simulink model "VCU_CS75_12_30_test"  (R2014a)
settings: Solver=FixedStepDiscrete  StartTime=0.0  StopTime=25  FixedStep=0.0005  RelTol=1e-3
InitFcn:
  | PID_canshu
values from neighbouring files (symbols this model uses):
  D1 = ecucoder_cal(D1)    [PID_canshu.m]
  D2 = ecucoder_cal(D2)    [PID_canshu.m]
  D3 = ecucoder_cal(D3)    [PID_canshu.m]
  ErrorLimit = ecucoder_cal(ErrorLimit)    [PID_canshu.m]
  ErrorSumMax1 = ecucoder_cal(ErrorSumMax1)    [PID_canshu.m]
  ErrorSumMax2 = ecucoder_cal(ErrorSumMax2)    [PID_canshu.m]
  ErrorSumMax3 = ecucoder_cal(ErrorSumMax3)    [PID_canshu.m]
  I1 = ecucoder_cal(I1)    [PID_canshu.m]
  I2 = ecucoder_cal(I2)    [PID_canshu.m]
  I3 = ecucoder_cal(I3)    [PID_canshu.m]
  Limit1 = ecucoder_cal(Limit1)    [PID_canshu.m]
  Limit2 = ecucoder_cal(Limit2)    [PID_canshu.m]
  P1 = ecucoder_cal(P1)    [PID_canshu.m]
  P2 = ecucoder_cal(P2)    [PID_canshu.m]
  P3 = ecucoder_cal(P3)    [PID_canshu.m]
  T_buchang = ecucoder_cal(T_buchang)    [PID_canshu.m]
undefined symbols (not defined in the file or in its folder): ecucoder_acal, I_SW01_L, LaterlAngleCommand, LDW, RemoteAcclPosition
libraries: simulink x940, ec5744lib x41
(part 13 of 31)

== system VCU_CS75_12_30_test/长安CS75底盘程序，20ms一次/Input/CAN1_Rx/GW_3A2/ReceiveMessages/Subsystem ==
  input : Inport
  Enable : EnablePort
  Bus Creator : BusCreator  Inputs=27
  GW_3A1 : Subsystem
  Signal Conversion : SignalConversion
  GW_3A2 : Outport
  wires:
  input/1 -> GW_3A1/1(input)
  Bus Creator/1 -> Signal Conversion/1
  GW_3A1/1(EPS_TorqueAssistMode_Out) -> Bus Creator/1  "EPS_TorqueAssistMode"
  GW_3A1/2(EMS_RemindGear_Out) -> Bus Creator/2  "EMS_RemindGear"
  GW_3A1/3(TCU_FailureLamp_Out) -> Bus Creator/3  "TCU_FailureLamp"
  GW_3A1/4(ACC_ACCMode_Out) -> Bus Creator/4  "ACC_ACCMode"
  GW_3A1/5(TCU_WNTLamp_Out) -> Bus Creator/5  "TCU_WNTLamp"
  GW_3A1/6(TCU_PWRLamp_Out) -> Bus Creator/6  "TCU_PWRLamp"
  GW_3A1/7(SRS_LeftRearBuckleSwitchSts_Out) -> Bus Creator/7  "SRS_LeftRearBuckleSwitchSts"
  GW_3A1/8(SRS_MiddleRearBuckleSwitchSts_Out) -> Bus Creator/8  "SRS_MiddleRearBuckleSwitchSts"
  GW_3A1/9(SRS_RightRearBuckleSwitchSts_Out) -> Bus Creator/9  "SRS_RightRearBuckleSwitchSts"
  GW_3A1/10(EPB_TextDisplay_Out) -> Bus Creator/10  "EPB_TextDisplay"
  GW_3A1/11(ESP_ESPActiveStatus_Out) -> Bus Creator/11  "ESP_ESPActiveStatus"
  GW_3A1/12(ESP_ESPFunctionStatus_Out) -> Bus Creator/12  "ESP_ESPFunctionStatus"
  GW_3A1/13(ESP_EBDFailStatus_Out) -> Bus Creator/13  "ESP_EBDFailStatus"
  GW_3A1/14(EPS_EPSFailed_Out) -> Bus Creator/14  "EPS_EPSFailed"
  GW_3A1/15(EPB_FunctionLamp_Out) -> Bus Creator/15  "EPB_FunctionLamp"
  GW_3A1/16(EPB_SwitchPosition_Out) -> Bus Creator/16  "EPB_SwitchPosition"
  GW_3A1/17(EPB_SwitchPositionValid_Out) -> Bus Creator/17  "EPB_SwitchPositionValid"
  GW_3A1/18(ESP_HDC_STATUS_Out) -> Bus Creator/18  "ESP_HDC_STATUS"
  GW_3A1/19(ESP_AutoHoldAvailable_Out) -> Bus Creator/19  "ESP_AutoHoldAvailable"
  GW_3A1/20(ESP_HHC_Active_Out) -> Bus Creator/20  "ESP_HHC_Active"
  GW_3A1/21(ESP_AutoHoldActive_Out) -> Bus Creator/21  "ESP_AutoHoldActive"
  GW_3A1/22(ESP_HHC_Available_Out) -> Bus Creator/22  "ESP_HHC_Available"
  GW_3A1/23(TCU_GearForDisplay_Out) -> Bus Creator/23  "TCU_GearForDisplay"
  GW_3A1/24(ESP_HBBFunctionStatus_Out) -> Bus Creator/24  "ESP_HBBFunctionStatus"
  GW_3A1/25(TCU_GearIndication_Out) -> Bus Creator/25  "TCU_GearIndication"
  GW_3A1/26(TCU_ReqTranTempWarning_Out) -> Bus Creator/26  "TCU_ReqTranTempWarning"
  GW_3A1/27(EMS_RemindShiftGear_Out) -> Bus Creator/27  "EMS_RemindShiftGear"
  Signal Conversion/1 -> GW_3A2/1

== system VCU_CS75_12_30_test/长安CS75底盘程序，20ms一次/Input/CAN1_Rx/GW_567/ReceiveMessages/Subsystem ==
  input : Inport
  Enable : EnablePort
  Bus Creator : BusCreator  Inputs=5
  GW_2 : Subsystem
  Signal Conversion : SignalConversion
  GW_567 : Outport
  wires:
  Bus Creator/1 -> Signal Conversion/1
  input/1 -> GW_2/1(input)
  GW_2/1(HU_EnterTunnelInfo_Out) -> Bus Creator/1  "HU_EnterTunnelInfo"
  GW_2/2(HU_TunnelDistance_Out) -> Bus Creator/2  "HU_TunnelDistance"
  GW_2/3(HU_TunnelLength_Out) -> Bus Creator/3  "HU_TunnelLength"
  GW_2/4(HU_Byroad_Out) -> Bus Creator/4  "HU_Byroad"
  GW_2/5(HU_NavGuiganceStatus_Out) -> Bus Creator/5  "HU_NavGuiganceStatus"
  Signal Conversion/1 -> GW_567/1

== system VCU_CS75_12_30_test/长安CS75底盘程序，20ms一次/Input/CAN1_Rx/HU_GPS_500/ReceiveMessages/Subsystem ==
  input : Inport
  Enable : EnablePort
  Bus Creator : BusCreator  Inputs=1
  HU_GPS_1 : Subsystem
  Signal Conversion : SignalConversion
  HU_GPS_500 : Outport
  wires:
  input/1 -> HU_GPS_1/1(input)
  Bus Creator/1 -> Signal Conversion/1
  HU_GPS_1/1(GPSCurrentLocationValid_Out) -> Bus Creator/1  "GPSCurrentLocationValid"
  Signal Conversion/1 -> HU_GPS_500/1

== system VCU_CS75_12_30_test/长安CS75底盘程序，20ms一次/Input/CAN1_Rx/LAS_36E/ReceiveMessages/Subsystem ==
  input : Inport
  Enable : EnablePort
  Bus Creator : BusCreator  Inputs=7
  LAS_36E2 : Subsystem
  Signal Conversion : SignalConversion
  LAS_36E : Outport
  wires:
  Bus Creator/1 -> Signal Conversion/1
  input/1 -> LAS_36E2/1(input)
  LAS_36E2/1(LAS_RoadCurvatureFar_Out) -> Bus Creator/1  "LAS_RoadCurvatureFar"
  LAS_36E2/2(LAS_RoadCurvatureNear_Out) -> Bus Creator/2  "LAS_RoadCurvatureNear"
  LAS_36E2/3(LAS_LaneEquationC1_Out) -> Bus Creator/3  "LAS_LaneEquationC1"
  LAS_36E2/4(LAS_LaneEquationC3_Out) -> Bus Creator/4  "LAS_LaneEquationC3"
  LAS_36E2/5(LAS_RollingCounter_id36E_Out) -> Bus Creator/5  "LAS_RollingCounter_id36E"
  LAS_36E2/6(LAS_LaneEquationStatus_Out) -> Bus Creator/6  "LAS_LaneEquationStatus"
  LAS_36E2/7(LAS_CheckSum_id36E_Out) -> Bus Creator/7  "LAS_CheckSum_id36E"
  Signal Conversion/1 -> LAS_36E/1

== system VCU_CS75_12_30_test/长安CS75底盘程序，20ms一次/Input/CAN1_Rx/SAS_108/ReceiveMessages/Subsystem ==
  input : Inport
  Enable : EnablePort
  Bus Creator : BusCreator  Inputs=7
  SAS_2 : Subsystem
  Signal Conversion : SignalConversion
  SAS_108 : Outport
  wires:
  Bus Creator/1 -> Signal Conversion/1
  input/1 -> SAS_2/1(input)
  SAS_2/1(SAS_SteeringAngle_Out) -> Bus Creator/1  "SAS_SteeringAngle"
  SAS_2/2(SAS_SteeringAngleSpeed_Out) -> Bus Creator/2  "SAS_SteeringAngleSpeed"
  SAS_2/3(SAS_Calibrated_Out) -> Bus Creator/3  "SAS_Calibrated"
  SAS_2/4(SAS_SASFailure_Out) -> Bus Creator/4  "SAS_SASFailure"
  SAS_2/5(SAS_SteeringAngleValid_Out) -> Bus Creator/5  "SAS_SteeringAngleValid"
  SAS_2/6(SAS_RollingCounter_Out) -> Bus Creator/6  "SAS_RollingCounter"
  SAS_2/7(SAS_CRCCheck_Out) -> Bus Creator/7  "SAS_CRCCheck"
  Signal Conversion/1 -> SAS_108/1

== system VCU_CS75_12_30_test/长安CS75底盘程序，20ms一次/Input/CAN1_Rx/SCM_3B8/ReceiveMessages/Subsystem ==
  input : Inport
  Enable : EnablePort
  Bus Creator : BusCreator  Inputs=6
  SCM_3B2 : Subsystem
  Signal Conversion : SignalConversion
  SCM_3B8 : Outport
  wires:
  input/1 -> SCM_3B2/1(input)
  Bus Creator/1 -> Signal Conversion/1
  SCM_3B2/6(SCM_IACCOn_Out) -> Bus Creator/6  "SCM_IACCOn"
  SCM_3B2/5(SCM_TimeGap_Out) -> Bus Creator/5  "SCM_TimeGap"
  SCM_3B2/4(SCM_Speeddecrease_Out) -> Bus Creator/4  "SCM_Speeddecrease"
  SCM_3B2/3(SCM_Resume_Out) -> Bus Creator/3  "SCM_Resume"
  SCM_3B2/2(SCM_ACCCancel_Out) -> Bus Creator/2  "SCM_ACCCancel"
  SCM_3B2/1(SCM_ACCOn_Out) -> Bus Creator/1  "SCM_ACCOn"
  Signal Conversion/1 -> SCM_3B8/1

== system VCU_CS75_12_30_test/长安CS75底盘程序，20ms一次/Input/CAN1_Rx/SRS_005/ReceiveMessages/Subsystem ==
  input : Inport
  Enable : EnablePort
  Bus Creator : BusCreator  Inputs=2
  SRS_1 : Subsystem
  Signal Conversion : SignalConversion
  SRS_005 : Outport
  wires:
  Bus Creator/1 -> Signal Conversion/1
  input/1 -> SRS_1/1(input)
  SRS_1/1(SRS_DriverBuckleSwitchStatus_Out) -> Bus Creator/1  "SRS_DriverBuckleSwitchStatus"
  SRS_1/2(SRS_RollingCounter_Out) -> Bus Creator/2  "SRS_RollingCounter"
  Signal Conversion/1 -> SRS_005/1

== system VCU_CS75_12_30_test/长安CS75底盘程序，20ms一次/Input/CAN1_Rx/TCU_286/ReceiveMessages/Subsystem ==
  input : Inport
  Enable : EnablePort
  Bus Creator : BusCreator
  Signal Conversion : SignalConversion
  TCU_1 : Subsystem
  TCU_286 : Outport
  wires:
  input/1 -> TCU_1/1(input)
  Bus Creator/1 -> Signal Conversion/1
  TCU_1/1(TCU_ActualGear_Out) -> Bus Creator/1  "TCU_ActualGear"
  TCU_1/2(TCU_ShiftPositionValid_Out) -> Bus Creator/2  "TCU_ShiftPositionValid"
  TCU_1/3(TCU_ActualGearValid_Out) -> Bus Creator/3  "TCU_ActualGearValid"
  TCU_1/4(TCU_GearShiftPosition_Out) -> Bus Creator/4  "TCU_GearShiftPosition"
  Signal Conversion/1 -> TCU_286/1

== system VCU_CS75_12_30_test/长安CS75底盘程序，20ms一次/Input/DBC转化的messages（存底）/ReceiveMessages/EMS_205/EMS_CheckSum_205_Sub ==
  In1 : Inport
  Out1 : Outport
  wires:
  In1/1 -> Out1/1

== system VCU_CS75_12_30_test/长安CS75底盘程序，20ms一次/Input/DBC转化的messages（存底）/ReceiveMessages/EMS_205/EMS_ESPTorqReuestAvailability_Sub ==
  In1 : Inport
  Out1 : Outport
  wires:
  In1/1 -> Out1/1

== system VCU_CS75_12_30_test/长安CS75底盘程序，20ms一次/Input/DBC转化的messages（存底）/ReceiveMessages/EMS_205/EMS_FrictionalTorq_Sub ==
  In1 : Inport
  Out1 : Outport
  wires:
  In1/1 -> Out1/1

== system VCU_CS75_12_30_test/长安CS75底盘程序，20ms一次/Input/DBC转化的messages（存底）/ReceiveMessages/EMS_205/EMS_IndicatedDriverReqTorq_Sub ==
  In1 : Inport
  Out1 : Outport
  wires:
  In1/1 -> Out1/1

== system VCU_CS75_12_30_test/长安CS75底盘程序，20ms一次/Input/DBC转化的messages（存底）/ReceiveMessages/EMS_205/EMS_IndicatedRealEngTorq_Sub ==
  In1 : Inport
  Out1 : Outport
  wires:
  In1/1 -> Out1/1

== system VCU_CS75_12_30_test/长安CS75底盘程序，20ms一次/Input/DBC转化的messages（存底）/ReceiveMessages/EMS_205/EMS_RollingCounter_id205_Sub ==
  In1 : Inport
  Out1 : Outport
  wires:
  In1/1 -> Out1/1

== system VCU_CS75_12_30_test/长安CS75底盘程序，20ms一次/Input/DBC转化的messages（存底）/ReceiveMessages/EMS_205/EMS_TorqFailure_Sub ==
  In1 : Inport
  Out1 : Outport
  wires:
  In1/1 -> Out1/1

== system VCU_CS75_12_30_test/长安CS75底盘程序，20ms一次/Input/DBC转化的messages（存底）/ReceiveMessages1/EMS_255/EMS_AccPedal_Sub ==
  In1 : Inport
  Out1 : Outport
  wires:
  In1/1 -> Out1/1

== system VCU_CS75_12_30_test/长安CS75底盘程序，20ms一次/Input/DBC转化的messages（存底）/ReceiveMessages1/EMS_255/EMS_AccpedelError_Sub ==
  In1 : Inport
  Out1 : Outport
  wires:
  In1/1 -> Out1/1

== system VCU_CS75_12_30_test/长安CS75底盘程序，20ms一次/Input/DBC转化的messages（存底）/ReceiveMessages1/EMS_255/EMS_BrakePedalStatus_Sub ==
  In1 : Inport
  Out1 : Outport
  wires:
  In1/1 -> Out1/1

== system VCU_CS75_12_30_test/长安CS75底盘程序，20ms一次/Input/DBC转化的messages（存底）/ReceiveMessages1/EMS_255/EMS_CheckSum_255_Sub ==
  In1 : Inport
  Out1 : Outport
  wires:
  In1/1 -> Out1/1

== system VCU_CS75_12_30_test/长安CS75底盘程序，20ms一次/Input/DBC转化的messages（存底）/ReceiveMessages1/EMS_255/EMS_EngineSpeedError_Sub ==
  In1 : Inport
  Out1 : Outport
  wires:
  In1/1 -> Out1/1

== system VCU_CS75_12_30_test/长安CS75底盘程序，20ms一次/Input/DBC转化的messages（存底）/ReceiveMessages1/EMS_255/EMS_EngineSpeed_Sub ==
  In1 : Inport
  Out1 : Outport
  wires:
  In1/1 -> Out1/1

== system VCU_CS75_12_30_test/长安CS75底盘程序，20ms一次/Input/DBC转化的messages（存底）/ReceiveMessages1/EMS_255/EMS_RollingCounter_id255_Sub ==
  In1 : Inport
  Out1 : Outport
  wires:
  In1/1 -> Out1/1

== system VCU_CS75_12_30_test/长安CS75底盘程序，20ms一次/Input/DBC转化的messages（存底）/ReceiveMessages10/ESP_287/ESP_CheckSum_Sub ==
  In1 : Inport
  Out1 : Outport
  wires:
  In1/1 -> Out1/1

== system VCU_CS75_12_30_test/长安CS75底盘程序，20ms一次/Input/DBC转化的messages（存底）/ReceiveMessages10/ESP_287/ESP_HBBActiveStatus_Sub ==
  In1 : Inport
  Out1 : Outport
  wires:
  In1/1 -> Out1/1

== system VCU_CS75_12_30_test/长安CS75底盘程序，20ms一次/Input/DBC转化的messages（存底）/ReceiveMessages10/ESP_287/ESP_HBB_Status_Sub ==
  In1 : Inport
  Out1 : Outport
  wires:
  In1/1 -> Out1/1

== system VCU_CS75_12_30_test/长安CS75底盘程序，20ms一次/Input/DBC转化的messages（存底）/ReceiveMessages10/ESP_287/ESP_HDC_Status_Sub ==
  In1 : Inport
  Out1 : Outport
  wires:
  In1/1 -> Out1/1

== system VCU_CS75_12_30_test/长安CS75底盘程序，20ms一次/Input/DBC转化的messages（存底）/ReceiveMessages10/ESP_287/ESP_HHC_Available_Sub ==
  In1 : Inport
  Out1 : Outport
  wires:
  In1/1 -> Out1/1

== system VCU_CS75_12_30_test/长安CS75底盘程序，20ms一次/Input/DBC转化的messages（存底）/ReceiveMessages10/ESP_287/ESP_LatAcceleration_Sub ==
  In1 : Inport
  Out1 : Outport
  wires:
  In1/1 -> Out1/1

== system VCU_CS75_12_30_test/长安CS75底盘程序，20ms一次/Input/DBC转化的messages（存底）/ReceiveMessages10/ESP_287/ESP_LongAccelValid_Sub ==
  In1 : Inport
  Out1 : Outport
  wires:
  In1/1 -> Out1/1

== system VCU_CS75_12_30_test/长安CS75底盘程序，20ms一次/Input/DBC转化的messages（存底）/ReceiveMessages10/ESP_287/ESP_LongAcceleration_Sub ==
  In1 : Inport
  Out1 : Outport
  wires:
  In1/1 -> Out1/1

== system VCU_CS75_12_30_test/长安CS75底盘程序，20ms一次/Input/DBC转化的messages（存底）/ReceiveMessages10/ESP_287/ESP_RollingCounter_Sub ==
  In1 : Inport
  Out1 : Outport
  wires:
  In1/1 -> Out1/1

== system VCU_CS75_12_30_test/长安CS75底盘程序，20ms一次/Input/DBC转化的messages（存底）/ReceiveMessages10/ESP_287/ESP_TODFastOpenRequest_Sub ==
  In1 : Inport
  Out1 : Outport
  wires:
  In1/1 -> Out1/1

== system VCU_CS75_12_30_test/长安CS75底盘程序，20ms一次/Input/DBC转化的messages（存底）/ReceiveMessages10/ESP_287/ESP_TODTorqueMaxLimit_Sub ==
  In1 : Inport
  Out1 : Outport
  wires:
  In1/1 -> Out1/1

== system VCU_CS75_12_30_test/长安CS75底盘程序，20ms一次/Input/DBC转化的messages（存底）/ReceiveMessages10/ESP_287/ESP_YawRate_Status_Sub ==
  In1 : Inport
  Out1 : Outport
  wires:
  In1/1 -> Out1/1

== system VCU_CS75_12_30_test/长安CS75底盘程序，20ms一次/Input/DBC转化的messages（存底）/ReceiveMessages10/ESP_287/ESP_YawRate_Sub ==
  In1 : Inport
  Out1 : Outport
  wires:
  In1/1 -> Out1/1

== system VCU_CS75_12_30_test/长安CS75底盘程序，20ms一次/Input/DBC转化的messages（存底）/ReceiveMessages11/HU_AEBSetting_551/HU_AEBOnOffSetting_Sub ==
  In1 : Inport
  Out1 : Outport
  wires:
  In1/1 -> Out1/1

== system VCU_CS75_12_30_test/长安CS75底盘程序，20ms一次/Input/DBC转化的messages（存底）/ReceiveMessages11/HU_AEBSetting_551/HU_FCWSetting_Sub ==
  In1 : Inport
  Out1 : Outport
  wires:
  In1/1 -> Out1/1

== system VCU_CS75_12_30_test/长安CS75底盘程序，20ms一次/Input/DBC转化的messages（存底）/ReceiveMessages11/HU_AEBSetting_551/HU_LCASetting_Sub ==
  In1 : Inport
  Out1 : Outport
  wires:
  In1/1 -> Out1/1

== system VCU_CS75_12_30_test/长安CS75底盘程序，20ms一次/Input/DBC转化的messages（存底）/ReceiveMessages12/HU_LASSetting_0x541/HU_AudioWarningEnable_Sub ==
  In1 : Inport
  Out1 : Outport
  wires:
  In1/1 -> Out1/1

== system VCU_CS75_12_30_test/长安CS75底盘程序，20ms一次/Input/DBC转化的messages（存底）/ReceiveMessages12/HU_LASSetting_0x541/HU_BSD_LCAEnable_Sub ==
  In1 : Inport
  Out1 : Outport
  wires:
  In1/1 -> Out1/1

== system VCU_CS75_12_30_test/长安CS75底盘程序，20ms一次/Input/DBC转化的messages（存底）/ReceiveMessages12/HU_LASSetting_0x541/HU_CTAEnable_Sub ==
  In1 : Inport
  Out1 : Outport
  wires:
  In1/1 -> Out1/1

== system VCU_CS75_12_30_test/长安CS75底盘程序，20ms一次/Input/DBC转化的messages（存底）/ReceiveMessages12/HU_LASSetting_0x541/HU_DSMMemoryPositionFeedback_Sub ==
  In1 : Inport
  Out1 : Outport
  wires:
  In1/1 -> Out1/1

== system VCU_CS75_12_30_test/长安CS75底盘程序，20ms一次/Input/DBC转化的messages（存底）/ReceiveMessages12/HU_LASSetting_0x541/HU_DVRBrowseCommand_Sub ==
  In1 : Inport
  Out1 : Outport
  wires:
  In1/1 -> Out1/1

== system VCU_CS75_12_30_test/长安CS75底盘程序，20ms一次/Input/DBC转化的messages（存底）/ReceiveMessages12/HU_LASSetting_0x541/HU_HMAEnable_Sub ==
  In1 : Inport
  Out1 : Outport
  wires:
  In1/1 -> Out1/1

== system VCU_CS75_12_30_test/长安CS75底盘程序，20ms一次/Input/DBC转化的messages（存底）/ReceiveMessages12/HU_LASSetting_0x541/HU_IACCEnable_Sub ==
  In1 : Inport
  Out1 : Outport
  wires:
  In1/1 -> Out1/1

== system VCU_CS75_12_30_test/长安CS75底盘程序，20ms一次/Input/DBC转化的messages（存底）/ReceiveMessages12/HU_LASSetting_0x541/HU_LASModeSelection_Sub ==
  In1 : Inport
  Out1 : Outport
  wires:
  In1/1 -> Out1/1

== system VCU_CS75_12_30_test/长安CS75底盘程序，20ms一次/Input/DBC转化的messages（存底）/ReceiveMessages12/HU_LASSetting_0x541/HU_LASWarningModeSelection_Sub ==
  In1 : Inport
  Out1 : Outport
  wires:
  In1/1 -> Out1/1

== system VCU_CS75_12_30_test/长安CS75底盘程序，20ms一次/Input/DBC转化的messages（存底）/ReceiveMessages12/HU_LASSetting_0x541/HU_LCATTCSetting_Sub ==
  In1 : Inport
  Out1 : Outport
  wires:
  In1/1 -> Out1/1

== system VCU_CS75_12_30_test/长安CS75底盘程序，20ms一次/Input/DBC转化的messages（存底）/ReceiveMessages12/HU_LASSetting_0x541/HU_LDWShakeLev_Sub ==
  In1 : Inport
  Out1 : Outport
  wires:
  In1/1 -> Out1/1

== system VCU_CS75_12_30_test/长安CS75底盘程序，20ms一次/Input/DBC转化的messages（存底）/ReceiveMessages12/HU_LASSetting_0x541/HU_LdwSensitivity_Sub ==
  In1 : Inport
  Out1 : Outport
  wires:
  In1/1 -> Out1/1

== system VCU_CS75_12_30_test/长安CS75底盘程序，20ms一次/Input/DBC转化的messages（存底）/ReceiveMessages12/HU_LASSetting_0x541/HU_LockCtrlEnable_Sub ==
  In1 : Inport
  Out1 : Outport
  wires:
  In1/1 -> Out1/1

== system VCU_CS75_12_30_test/长安CS75底盘程序，20ms一次/Input/DBC转化的messages（存底）/ReceiveMessages12/HU_LASSetting_0x541/HU_ObstacleSafeDistanceSet_Sub ==
  In1 : Inport
  Out1 : Outport
  wires:
  In1/1 -> Out1/1

== system VCU_CS75_12_30_test/长安CS75底盘程序，20ms一次/Input/DBC转化的messages（存底）/ReceiveMessages12/HU_LASSetting_0x541/HU_OverspeedSoundWarEnable_Sub ==
  In1 : Inport
  Out1 : Outport
  wires:
  In1/1 -> Out1/1

== system VCU_CS75_12_30_test/长安CS75底盘程序，20ms一次/Input/DBC转化的messages（存底）/ReceiveMessages12/HU_LASSetting_0x541/HU_OverspeedWarningEnable_Sub ==
  In1 : Inport
  Out1 : Outport
  wires:
  In1/1 -> Out1/1

== system VCU_CS75_12_30_test/长安CS75底盘程序，20ms一次/Input/DBC转化的messages（存底）/ReceiveMessages12/HU_LASSetting_0x541/HU_OverspeedWarningOffset_Sub ==
  In1 : Inport
  Out1 : Outport
  wires:
  In1/1 -> Out1/1

== system VCU_CS75_12_30_test/长安CS75底盘程序，20ms一次/Input/DBC转化的messages（存底）/ReceiveMessages12/HU_LASSetting_0x541/HU_ParkingConfirm_Sub ==
  In1 : Inport
  Out1 : Outport
  wires:
  In1/1 -> Out1/1

== system VCU_CS75_12_30_test/长安CS75底盘程序，20ms一次/Input/DBC转化的messages（存底）/ReceiveMessages12/HU_LASSetting_0x541/HU_ParkingResume_Sub ==
  In1 : Inport
  Out1 : Outport
  wires:
  In1/1 -> Out1/1

== system VCU_CS75_12_30_test/长安CS75底盘程序，20ms一次/Input/DBC转化的messages（存底）/ReceiveMessages12/HU_LASSetting_0x541/HU_RCWEnable_Sub ==
  In1 : Inport
  Out1 : Outport
  wires:
  In1/1 -> Out1/1

== system VCU_CS75_12_30_test/长安CS75底盘程序，20ms一次/Input/DBC转化的messages（存底）/ReceiveMessages12/HU_LASSetting_0x541/HU_RCWSoundEnable_Sub ==
  In1 : Inport
  Out1 : Outport
  wires:
  In1/1 -> Out1/1

== system VCU_CS75_12_30_test/长安CS75底盘程序，20ms一次/Input/DBC转化的messages（存底）/ReceiveMessages12/HU_LASSetting_0x541/HU_RemoteDistanceSet_Sub ==
  In1 : Inport
  Out1 : Outport
  wires:
  In1/1 -> Out1/1

== system VCU_CS75_12_30_test/长安CS75底盘程序，20ms一次/Input/DBC转化的messages（存底）/ReceiveMessages12/HU_LASSetting_0x541/HU_SEWEnable_Sub ==
  In1 : Inport
  Out1 : Outport
  wires:
  In1/1 -> Out1/1

== system VCU_CS75_12_30_test/长安CS75底盘程序，20ms一次/Input/DBC转化的messages（存底）/ReceiveMessages12/HU_LASSetting_0x541/HU_SLASwitch_Sub ==
  In1 : Inport
  Out1 : Outport
  wires:
  In1/1 -> Out1/1

== system VCU_CS75_12_30_test/长安CS75底盘程序，20ms一次/Input/DBC转化的messages（存底）/ReceiveMessages12/HU_LASSetting_0x541/HU_Uls_BSD_Activation_Sub ==
  In1 : Inport
  Out1 : Outport
  wires:
  In1/1 -> Out1/1

== system VCU_CS75_12_30_test/长安CS75底盘程序，20ms一次/Input/DBC转化的messages（存底）/ReceiveMessages12/HU_LASSetting_0x541/HU_Uls_FKP_Activation_Sub ==
  In1 : Inport
  Out1 : Outport
  wires:
  In1/1 -> Out1/1

== system VCU_CS75_12_30_test/长安CS75底盘程序，20ms一次/Input/DBC转化的messages（存底）/ReceiveMessages13/SAS_108/SAS_CRCCheck_Sub ==
  In1 : Inport
  Out1 : Outport
  wires:
  In1/1 -> Out1/1

== system VCU_CS75_12_30_test/长安CS75底盘程序，20ms一次/Input/DBC转化的messages（存底）/ReceiveMessages13/SAS_108/SAS_Calibrated_Sub ==
  In1 : Inport
  Out1 : Outport
  wires:
  In1/1 -> Out1/1

== system VCU_CS75_12_30_test/长安CS75底盘程序，20ms一次/Input/DBC转化的messages（存底）/ReceiveMessages13/SAS_108/SAS_RollingCounter_Sub ==
  In1 : Inport
  Out1 : Outport
  wires:
  In1/1 -> Out1/1

== system VCU_CS75_12_30_test/长安CS75底盘程序，20ms一次/Input/DBC转化的messages（存底）/ReceiveMessages13/SAS_108/SAS_SASFailure_Sub ==
  In1 : Inport
  Out1 : Outport
  wires:
  In1/1 -> Out1/1

== system VCU_CS75_12_30_test/长安CS75底盘程序，20ms一次/Input/DBC转化的messages（存底）/ReceiveMessages13/SAS_108/SAS_SteeringAngleSpeed_Sub ==
  In1 : Inport
  Out1 : Outport
  wires:
  In1/1 -> Out1/1

== system VCU_CS75_12_30_test/长安CS75底盘程序，20ms一次/Input/DBC转化的messages（存底）/ReceiveMessages13/SAS_108/SAS_SteeringAngleValid_Sub ==
  In1 : Inport
  Out1 : Outport
  wires:
  In1/1 -> Out1/1

== system VCU_CS75_12_30_test/长安CS75底盘程序，20ms一次/Input/DBC转化的messages（存底）/ReceiveMessages13/SAS_108/SAS_SteeringAngle_Sub ==
  In1 : Inport
  Out1 : Outport
  wires:
  In1/1 -> Out1/1

== system VCU_CS75_12_30_test/长安CS75底盘程序，20ms一次/Input/DBC转化的messages（存底）/ReceiveMessages14/SCM_3B8/SCM_ACCCancel_Sub ==
  In1 : Inport
  Out1 : Outport
  wires:
  In1/1 -> Out1/1

== system VCU_CS75_12_30_test/长安CS75底盘程序，20ms一次/Input/DBC转化的messages（存底）/ReceiveMessages14/SCM_3B8/SCM_ACCOn_Sub ==
  In1 : Inport
  Out1 : Outport
  wires:
  In1/1 -> Out1/1

== system VCU_CS75_12_30_test/长安CS75底盘程序，20ms一次/Input/DBC转化的messages（存底）/ReceiveMessages14/SCM_3B8/SCM_IACCOn_Sub ==
  In1 : Inport
  Out1 : Outport
  wires:
  In1/1 -> Out1/1

== system VCU_CS75_12_30_test/长安CS75底盘程序，20ms一次/Input/DBC转化的messages（存底）/ReceiveMessages14/SCM_3B8/SCM_Resume_Sub ==
  In1 : Inport
  Out1 : Outport
  wires:
  In1/1 -> Out1/1

== system VCU_CS75_12_30_test/长安CS75底盘程序，20ms一次/Input/DBC转化的messages（存底）/ReceiveMessages14/SCM_3B8/SCM_Speeddecrease_Sub ==
  In1 : Inport
  Out1 : Outport
  wires:
  In1/1 -> Out1/1

== system VCU_CS75_12_30_test/长安CS75底盘程序，20ms一次/Input/DBC转化的messages（存底）/ReceiveMessages14/SCM_3B8/SCM_TimeGap_Sub ==
  In1 : Inport
  Out1 : Outport
  wires:
  In1/1 -> Out1/1

== system VCU_CS75_12_30_test/长安CS75底盘程序，20ms一次/Input/DBC转化的messages（存底）/ReceiveMessages15/SRS_005/SRS_DriverBuckleSwitchStatus_Sub ==
  In1 : Inport
  Out1 : Outport
  wires:
  In1/1 -> Out1/1

== system VCU_CS75_12_30_test/长安CS75底盘程序，20ms一次/Input/DBC转化的messages（存底）/ReceiveMessages15/SRS_005/SRS_RollingCounter_Sub ==
  In1 : Inport
  Out1 : Outport
  wires:
  In1/1 -> Out1/1

== system VCU_CS75_12_30_test/长安CS75底盘程序，20ms一次/Input/DBC转化的messages（存底）/ReceiveMessages16/TCU_286/TCU_ActualGearValid_Sub ==
  In1 : Inport
  Out1 : Outport
  wires:
  In1/1 -> Out1/1

== system VCU_CS75_12_30_test/长安CS75底盘程序，20ms一次/Input/DBC转化的messages（存底）/ReceiveMessages16/TCU_286/TCU_ActualGear_Sub ==
  In1 : Inport
  Out1 : Outport
  wires:
  In1/1 -> Out1/1

== system VCU_CS75_12_30_test/长安CS75底盘程序，20ms一次/Input/DBC转化的messages（存底）/ReceiveMessages16/TCU_286/TCU_GearShiftPosition_Sub ==
  In1 : Inport
  Out1 : Outport
  wires:
  In1/1 -> Out1/1

== system VCU_CS75_12_30_test/长安CS75底盘程序，20ms一次/Input/DBC转化的messages（存底）/ReceiveMessages16/TCU_286/TCU_ShiftPositionValid_Sub ==
  In1 : Inport
  Out1 : Outport
  wires:
  In1/1 -> Out1/1

== system VCU_CS75_12_30_test/长安CS75底盘程序，20ms一次/Input/DBC转化的messages（存底）/ReceiveMessages17/BCM_288/BCM_BuzzerWarningMode_Sub ==
  In1 : Inport
  Out1 : Outport
  wires:
  In1/1 -> Out1/1

== system VCU_CS75_12_30_test/长安CS75底盘程序，20ms一次/Input/DBC转化的messages（存底）/ReceiveMessages17/BCM_288/BCM_DriverDoorLockStatus_Sub ==
  In1 : Inport
  Out1 : Outport
  wires:
  In1/1 -> Out1/1

== system VCU_CS75_12_30_test/长安CS75底盘程序，20ms一次/Input/DBC转化的messages（存底）/ReceiveMessages17/BCM_288/BCM_DriverDoorStatus_Sub ==
  In1 : Inport
  Out1 : Outport
  wires:
  In1/1 -> Out1/1

== system VCU_CS75_12_30_test/长安CS75底盘程序，20ms一次/Input/DBC转化的messages（存底）/ReceiveMessages17/BCM_288/BCM_FrontWashStatus_Sub ==
  In1 : Inport
  Out1 : Outport
  wires:
  In1/1 -> Out1/1

== system VCU_CS75_12_30_test/长安CS75底盘程序，20ms一次/Input/DBC转化的messages（存底）/ReceiveMessages17/BCM_288/BCM_FrontWiperStatus_Sub ==
  In1 : Inport
  Out1 : Outport
  wires:
  In1/1 -> Out1/1

== system VCU_CS75_12_30_test/长安CS75底盘程序，20ms一次/Input/DBC转化的messages（存底）/ReceiveMessages17/BCM_288/BCM_HoodStatus_Sub ==
  In1 : Inport
  Out1 : Outport
  wires:
  In1/1 -> Out1/1

== system VCU_CS75_12_30_test/长安CS75底盘程序，20ms一次/Input/DBC转化的messages（存底）/ReceiveMessages17/BCM_288/BCM_LatchOverheatProtect_Sub ==
  In1 : Inport
  Out1 : Outport
  wires:
  In1/1 -> Out1/1

== system VCU_CS75_12_30_test/长安CS75底盘程序，20ms一次/Input/DBC转化的messages（存底）/ReceiveMessages17/BCM_288/BCM_LeftRearDoorStatus_Sub ==
  In1 : Inport
  Out1 : Outport
  wires:
  In1/1 -> Out1/1

== system VCU_CS75_12_30_test/长安CS75底盘程序，20ms一次/Input/DBC转化的messages（存底）/ReceiveMessages17/BCM_288/BCM_PassengerDoorLockStatus_Sub ==
  In1 : Inport
  Out1 : Outport
  wires:
  In1/1 -> Out1/1

== system VCU_CS75_12_30_test/长安CS75底盘程序，20ms一次/Input/DBC转化的messages（存底）/ReceiveMessages17/BCM_288/BCM_PassengerDoorStatus_Sub ==
  In1 : Inport
  Out1 : Outport
  wires:
  In1/1 -> Out1/1

== system VCU_CS75_12_30_test/长安CS75底盘程序，20ms一次/Input/DBC转化的messages（存底）/ReceiveMessages17/BCM_288/BCM_PowerStatusFeedback_Sub ==
  In1 : Inport
  Out1 : Outport
  wires:
  In1/1 -> Out1/1

== system VCU_CS75_12_30_test/长安CS75底盘程序，20ms一次/Input/DBC转化的messages（存底）/ReceiveMessages17/BCM_288/BCM_RearWiperStatus_Sub ==
  In1 : Inport
  Out1 : Outport
  wires:
  In1/1 -> Out1/1

== system VCU_CS75_12_30_test/长安CS75底盘程序，20ms一次/Input/DBC转化的messages（存底）/ReceiveMessages17/BCM_288/BCM_ReversePosition_Sub ==
  In1 : Inport
  Out1 : Outport
  wires:
  In1/1 -> Out1/1

== system VCU_CS75_12_30_test/长安CS75底盘程序，20ms一次/Input/DBC转化的messages（存底）/ReceiveMessages17/BCM_288/BCM_RightRearDoorStatus_Sub ==
  In1 : Inport
  Out1 : Outport
  wires:
  In1/1 -> Out1/1

== system VCU_CS75_12_30_test/长安CS75底盘程序，20ms一次/Input/DBC转化的messages（存底）/ReceiveMessages17/BCM_288/BCM_SystemFailureFlag_Sub ==
  In1 : Inport
  Out1 : Outport
  wires:
  In1/1 -> Out1/1

== system VCU_CS75_12_30_test/长安CS75底盘程序，20ms一次/Input/DBC转化的messages（存底）/ReceiveMessages17/BCM_288/BCM_TrunkDoorStatus_Sub ==
  In1 : Inport
  Out1 : Outport
  wires:
  In1/1 -> Out1/1

== system VCU_CS75_12_30_test/长安CS75底盘程序，20ms一次/Input/DBC转化的messages（存底）/ReceiveMessages17/BCM_288/BCM_TurnIndicatorLeft_Sub ==
  In1 : Inport
  Out1 : Outport
  wires:
  In1/1 -> Out1/1

== system VCU_CS75_12_30_test/长安CS75底盘程序，20ms一次/Input/DBC转化的messages（存底）/ReceiveMessages17/BCM_288/BCM_TurnIndicatorRight_Sub ==
  In1 : Inport
  Out1 : Outport
  wires:
  In1/1 -> Out1/1

== system VCU_CS75_12_30_test/长安CS75底盘程序，20ms一次/Input/DBC转化的messages（存底）/ReceiveMessages17/BCM_288/BCM_TurnLightSwitchSts_Sub ==
  In1 : Inport
  Out1 : Outport
  wires:
  In1/1 -> Out1/1

== system VCU_CS75_12_30_test/长安CS75底盘程序，20ms一次/Input/DBC转化的messages（存底）/ReceiveMessages17/BCM_288/BCM_emergencylightstatus_Sub ==
  In1 : Inport
  Out1 : Outport
  wires:
  In1/1 -> Out1/1

== system VCU_CS75_12_30_test/长安CS75底盘程序，20ms一次/Input/DBC转化的messages（存底）/ReceiveMessages18/BCM_328/LCM_DRLSts_Sub ==
  In1 : Inport
  Out1 : Outport
  wires:
  In1/1 -> Out1/1

== system VCU_CS75_12_30_test/长安CS75底盘程序，20ms一次/Input/DBC转化的messages（存底）/ReceiveMessages18/BCM_328/LCM_DriveMode_Sub ==
  In1 : Inport
  Out1 : Outport
  wires:
  In1/1 -> Out1/1

== system VCU_CS75_12_30_test/长安CS75底盘程序，20ms一次/Input/DBC转化的messages（存底）/ReceiveMessages18/BCM_328/LCM_LASSwitch_Sub ==
  In1 : Inport
  Out1 : Outport
  wires:
  In1/1 -> Out1/1

== system VCU_CS75_12_30_test/长安CS75底盘程序，20ms一次/Input/DBC转化的messages（存底）/ReceiveMessages18/BCM_328/LCM_RearLeftTuningLightFaultSts_Sub ==
  In1 : Inport
  Out1 : Outport
  wires:
  In1/1 -> Out1/1

== system VCU_CS75_12_30_test/长安CS75底盘程序，20ms一次/Input/DBC转化的messages（存底）/ReceiveMessages18/BCM_328/LCM_RearRightTuningLightFaultSts_Sub ==
  In1 : Inport
  Out1 : Outport
  wires:
  In1/1 -> Out1/1

== system VCU_CS75_12_30_test/长安CS75底盘程序，20ms一次/Input/DBC转化的messages（存底）/ReceiveMessages18/BCM_328/LCM_ReverseLightSts_Sub ==
  In1 : Inport
  Out1 : Outport
  wires:
  In1/1 -> Out1/1

== system VCU_CS75_12_30_test/长安CS75底盘程序，20ms一次/Input/DBC转化的messages（存底）/ReceiveMessages19/BCM_348/BCM_DriveMode_Sub ==
  In1 : Inport
  Out1 : Outport
  wires:
  In1/1 -> Out1/1

== system VCU_CS75_12_30_test/长安CS75底盘程序，20ms一次/Input/DBC转化的messages（存底）/ReceiveMessages19/BCM_348/BCM_LockSignal_Sub ==
  In1 : Inport
  Out1 : Outport
  wires:
  In1/1 -> Out1/1

== system VCU_CS75_12_30_test/长安CS75底盘程序，20ms一次/Input/DBC转化的messages（存底）/ReceiveMessages19/BCM_348/BCM_UnlockSignal_Sub ==
  In1 : Inport
  Out1 : Outport
  wires:
  In1/1 -> Out1/1

== system VCU_CS75_12_30_test/长安CS75底盘程序，20ms一次/Input/DBC转化的messages（存底）/ReceiveMessages2/EMS_265/EMS_EngineStatus_Sub ==
  In1 : Inport
  Out1 : Outport
  wires:
  In1/1 -> Out1/1

== system VCU_CS75_12_30_test/长安CS75底盘程序，20ms一次/Input/DBC转化的messages（存底）/ReceiveMessages2/EMS_265/EMS_FullLoadIndicatedTorq_Sub ==
  In1 : Inport
  Out1 : Outport
  wires:
  In1/1 -> Out1/1

== system VCU_CS75_12_30_test/长安CS75底盘程序，20ms一次/Input/DBC转化的messages（存底）/ReceiveMessages2/EMS_265/EMS_RollingCounter_id265_Sub ==
  In1 : Inport
  Out1 : Outport
  wires:
  In1/1 -> Out1/1

== system VCU_CS75_12_30_test/长安CS75底盘程序，20ms一次/Input/DBC转化的messages（存底）/ReceiveMessages2/EMS_265/EMS_TorqueConstant_Sub ==
  In1 : Inport
  Out1 : Outport
  wires:
  In1/1 -> Out1/1

== system VCU_CS75_12_30_test/长安CS75底盘程序，20ms一次/Input/DBC转化的messages（存底）/ReceiveMessages20/BCM_3DF/BCM_AmbientLightColorFeedback_Sub ==
  In1 : Inport
  Out1 : Outport
  wires:
  In1/1 -> Out1/1

== system VCU_CS75_12_30_test/长安CS75底盘程序，20ms一次/Input/DBC转化的messages（存底）/ReceiveMessages20/BCM_3DF/BCM_CRC_Checksum_Sub ==
  In1 : Inport
  Out1 : Outport
  wires:
  In1/1 -> Out1/1

== system VCU_CS75_12_30_test/长安CS75底盘程序，20ms一次/Input/DBC转化的messages（存底）/ReceiveMessages20/BCM_3DF/BCM_DriveModeFeedback_Sub ==
  In1 : Inport
  Out1 : Outport
  wires:
  In1/1 -> Out1/1

== system VCU_CS75_12_30_test/长安CS75底盘程序，20ms一次/Input/DBC转化的messages（存底）/ReceiveMessages20/BCM_3DF/BCM_DriveModeStatus_Sub ==
  In1 : Inport
  Out1 : Outport
  wires:
  In1/1 -> Out1/1

== system VCU_CS75_12_30_test/长安CS75底盘程序，20ms一次/Input/DBC转化的messages（存底）/ReceiveMessages20/BCM_3DF/BCM_DriveMode_Sub ==
  In1 : Inport
  Out1 : Outport
  wires:
  In1/1 -> Out1/1

== system VCU_CS75_12_30_test/长安CS75底盘程序，20ms一次/Input/DBC转化的messages（存底）/ReceiveMessages20/BCM_3DF/BCM_EPSTorqueModeFeedback_Sub ==
  In1 : Inport
  Out1 : Outport
  wires:
  In1/1 -> Out1/1

== system VCU_CS75_12_30_test/长安CS75底盘程序，20ms一次/Input/DBC转化的messages（存底）/ReceiveMessages20/BCM_3DF/BCM_EPSTorqueMode_Sub ==
  In1 : Inport
  Out1 : Outport
  wires:
  In1/1 -> Out1/1

== system VCU_CS75_12_30_test/长安CS75底盘程序，20ms一次/Input/DBC转化的messages（存底）/ReceiveMessages20/BCM_3DF/BCM_RollingCounter_Sub ==
  In1 : Inport
  Out1 : Outport
  wires:
  In1/1 -> Out1/1

== system VCU_CS75_12_30_test/长安CS75底盘程序，20ms一次/Input/DBC转化的messages（存底）/ReceiveMessages21/GW_20B/EMS_BrakePedalStatus_Sub ==
  In1 : Inport
  Out1 : Outport
  wires:
  In1/1 -> Out1/1

== system VCU_CS75_12_30_test/长安CS75底盘程序，20ms一次/Input/DBC转化的messages（存底）/ReceiveMessages21/GW_20B/EMS_EngineStartupEnd_Sub ==
  In1 : Inport
  Out1 : Outport
  wires:
  In1/1 -> Out1/1

== system VCU_CS75_12_30_test/长安CS75底盘程序，20ms一次/Input/DBC转化的messages（存底）/ReceiveMessages21/GW_20B/EMS_EngineStatus_Sub ==
  In1 : Inport
  Out1 : Outport
  wires:
  In1/1 -> Out1/1

== system VCU_CS75_12_30_test/长安CS75底盘程序，20ms一次/Input/DBC转化的messages（存底）/ReceiveMessages21/GW_20B/EPB_BrakeLightOnRequest_Sub ==
  In1 : Inport
  Out1 : Outport
  wires:
  In1/1 -> Out1/1

== system VCU_CS75_12_30_test/长安CS75底盘程序，20ms一次/Input/DBC转化的messages（存底）/ReceiveMessages21/GW_20B/EPB_Status_Sub ==
  In1 : Inport
  Out1 : Outport
  wires:
  In1/1 -> Out1/1

== system VCU_CS75_12_30_test/长安CS75底盘程序，20ms一次/Input/DBC转化的messages（存底）/ReceiveMessages21/GW_20B/SAS_SteeringAngleValid_Sub ==
  In1 : Inport
  Out1 : Outport
  wires:
  In1/1 -> Out1/1

== system VCU_CS75_12_30_test/长安CS75底盘程序，20ms一次/Input/DBC转化的messages（存底）/ReceiveMessages21/GW_20B/SAS_SteeringAngle_Sub ==
  In1 : Inport
  Out1 : Outport
  wires:
  In1/1 -> Out1/1

== system VCU_CS75_12_30_test/长安CS75底盘程序，20ms一次/Input/DBC转化的messages（存底）/ReceiveMessages21/GW_20B/TCU_GearShiftPositon_Sub ==
  In1 : Inport
  Out1 : Outport
  wires:
  In1/1 -> Out1/1

== system VCU_CS75_12_30_test/长安CS75底盘程序，20ms一次/Input/DBC转化的messages（存底）/ReceiveMessages21/GW_20B/TCU_ShiftPostionValid_Sub ==
  In1 : Inport
  Out1 : Outport
  wires:
  In1/1 -> Out1/1

== system VCU_CS75_12_30_test/长安CS75底盘程序，20ms一次/Input/DBC转化的messages（存底）/ReceiveMessages22/GW_332/EMS_EngineSpeed_Sub ==
  In1 : Inport
  Out1 : Outport
  wires:
  In1/1 -> Out1/1

== system VCU_CS75_12_30_test/长安CS75底盘程序，20ms一次/Input/DBC转化的messages（存底）/ReceiveMessages22/GW_332/SAS_SASFailure_Sub ==
  In1 : Inport
  Out1 : Outport
  wires:
  In1/1 -> Out1/1

== system VCU_CS75_12_30_test/长安CS75底盘程序，20ms一次/Input/DBC转化的messages（存底）/ReceiveMessages22/GW_332/SRS_DriverBuckleSwitchStatus_Sub ==
  In1 : Inport
  Out1 : Outport
  wires:
  In1/1 -> Out1/1

== system VCU_CS75_12_30_test/长安CS75底盘程序，20ms一次/Input/DBC转化的messages（存底）/ReceiveMessages22/GW_332/SRS_PassengerBuckleSwitchStatus_Sub ==
  In1 : Inport
  Out1 : Outport
  wires:
  In1/1 -> Out1/1

== system VCU_CS75_12_30_test/长安CS75底盘程序，20ms一次/Input/DBC转化的messages（存底）/ReceiveMessages23/GW_308/IP_TotalOdometer_Sub ==
  In1 : Inport
  Out1 : Outport
  wires:
  In1/1 -> Out1/1

== system VCU_CS75_12_30_test/长安CS75底盘程序，20ms一次/Input/DBC转化的messages（存底）/ReceiveMessages24/GW_376/EMS_ConditionIdle_Sub ==
  In1 : Inport
  Out1 : Outport
  wires:
  In1/1 -> Out1/1

== system VCU_CS75_12_30_test/长安CS75底盘程序，20ms一次/Input/DBC转化的messages（存底）/ReceiveMessages24/GW_376/EMS_EngineFuelCutOff_Sub ==
  In1 : Inport
  Out1 : Outport
  wires:
  In1/1 -> Out1/1

== system VCU_CS75_12_30_test/长安CS75底盘程序，20ms一次/Input/DBC转化的messages（存底）/ReceiveMessages24/GW_376/EMS_FrictionalTorq_Sub ==
  In1 : Inport
  Out1 : Outport
  wires:
  In1/1 -> Out1/1

== system VCU_CS75_12_30_test/长安CS75底盘程序，20ms一次/Input/DBC转化的messages（存底）/ReceiveMessages24/GW_376/EMS_TorqueConstant_Sub ==
  In1 : Inport
  Out1 : Outport
  wires:
  In1/1 -> Out1/1

== system VCU_CS75_12_30_test/长安CS75底盘程序，20ms一次/Input/DBC转化的messages（存底）/ReceiveMessages25/GW_3A2/ACC_ACCMode_Sub ==
  In1 : Inport
  Out1 : Outport
  wires:
  In1/1 -> Out1/1

== system VCU_CS75_12_30_test/长安CS75底盘程序，20ms一次/Input/DBC转化的messages（存底）/ReceiveMessages25/GW_3A2/EMS_RemindGear_Sub ==
  In1 : Inport
  Out1 : Outport
  wires:
  In1/1 -> Out1/1

== system VCU_CS75_12_30_test/长安CS75底盘程序，20ms一次/Input/DBC转化的messages（存底）/ReceiveMessages25/GW_3A2/EMS_RemindShiftGear_Sub ==
  In1 : Inport
  Out1 : Outport
  wires:
  In1/1 -> Out1/1

== system VCU_CS75_12_30_test/长安CS75底盘程序，20ms一次/Input/DBC转化的messages（存底）/ReceiveMessages25/GW_3A2/EPB_FunctionLamp_Sub ==
  In1 : Inport
  Out1 : Outport
  wires:
  In1/1 -> Out1/1

== system VCU_CS75_12_30_test/长安CS75底盘程序，20ms一次/Input/DBC转化的messages（存底）/ReceiveMessages25/GW_3A2/EPB_SwitchPositionValid_Sub ==
  In1 : Inport
  Out1 : Outport
  wires:
  In1/1 -> Out1/1

== system VCU_CS75_12_30_test/长安CS75底盘程序，20ms一次/Input/DBC转化的messages（存底）/ReceiveMessages25/GW_3A2/EPB_SwitchPosition_Sub ==
  In1 : Inport
  Out1 : Outport
  wires:
  In1/1 -> Out1/1

== system VCU_CS75_12_30_test/长安CS75底盘程序，20ms一次/Input/DBC转化的messages（存底）/ReceiveMessages25/GW_3A2/EPB_TextDisplay_Sub ==
  In1 : Inport
  Out1 : Outport
  wires:
  In1/1 -> Out1/1

== system VCU_CS75_12_30_test/长安CS75底盘程序，20ms一次/Input/DBC转化的messages（存底）/ReceiveMessages25/GW_3A2/EPS_EPSFailed_Sub ==
  In1 : Inport
  Out1 : Outport
  wires:
  In1/1 -> Out1/1

== system VCU_CS75_12_30_test/长安CS75底盘程序，20ms一次/Input/DBC转化的messages（存底）/ReceiveMessages25/GW_3A2/EPS_TorqueAssistMode_Sub ==
  In1 : Inport
  Out1 : Outport
  wires:
  In1/1 -> Out1/1

== system VCU_CS75_12_30_test/长安CS75底盘程序，20ms一次/Input/DBC转化的messages（存底）/ReceiveMessages25/GW_3A2/ESP_AutoHoldActive_Sub ==
  In1 : Inport
  Out1 : Outport
  wires:
  In1/1 -> Out1/1

== system VCU_CS75_12_30_test/长安CS75底盘程序，20ms一次/Input/DBC转化的messages（存底）/ReceiveMessages25/GW_3A2/ESP_AutoHoldAvailable_Sub ==
  In1 : Inport
  Out1 : Outport
  wires:
  In1/1 -> Out1/1

== system VCU_CS75_12_30_test/长安CS75底盘程序，20ms一次/Input/DBC转化的messages（存底）/ReceiveMessages25/GW_3A2/ESP_EBDFailStatus_Sub ==
  In1 : Inport
  Out1 : Outport
  wires:
  In1/1 -> Out1/1

== system VCU_CS75_12_30_test/长安CS75底盘程序，20ms一次/Input/DBC转化的messages（存底）/ReceiveMessages25/GW_3A2/ESP_ESPActiveStatus_Sub ==
  In1 : Inport
  Out1 : Outport
  wires:
  In1/1 -> Out1/1

== system VCU_CS75_12_30_test/长安CS75底盘程序，20ms一次/Input/DBC转化的messages（存底）/ReceiveMessages25/GW_3A2/ESP_ESPFunctionStatus_Sub ==
  In1 : Inport
  Out1 : Outport
  wires:
  In1/1 -> Out1/1

== system VCU_CS75_12_30_test/长安CS75底盘程序，20ms一次/Input/DBC转化的messages（存底）/ReceiveMessages25/GW_3A2/ESP_HBBFunctionStatus_Sub ==
  In1 : Inport
  Out1 : Outport
  wires:
  In1/1 -> Out1/1

== system VCU_CS75_12_30_test/长安CS75底盘程序，20ms一次/Input/DBC转化的messages（存底）/ReceiveMessages25/GW_3A2/ESP_HDC_STATUS_Sub ==
  In1 : Inport
  Out1 : Outport
  wires:
  In1/1 -> Out1/1

== system VCU_CS75_12_30_test/长安CS75底盘程序，20ms一次/Input/DBC转化的messages（存底）/ReceiveMessages25/GW_3A2/ESP_HHC_Active_Sub ==
  In1 : Inport
  Out1 : Outport
  wires:
  In1/1 -> Out1/1

== system VCU_CS75_12_30_test/长安CS75底盘程序，20ms一次/Input/DBC转化的messages（存底）/ReceiveMessages25/GW_3A2/ESP_HHC_Available_Sub ==
  In1 : Inport
  Out1 : Outport
  wires:
  In1/1 -> Out1/1

== system VCU_CS75_12_30_test/长安CS75底盘程序，20ms一次/Input/DBC转化的messages（存底）/ReceiveMessages25/GW_3A2/SRS_LeftRearBuckleSwitchSts_Sub ==
  In1 : Inport
  Out1 : Outport
  wires:
  In1/1 -> Out1/1

== system VCU_CS75_12_30_test/长安CS75底盘程序，20ms一次/Input/DBC转化的messages（存底）/ReceiveMessages25/GW_3A2/SRS_MiddleRearBuckleSwitchSts_Sub ==
  In1 : Inport
  Out1 : Outport
  wires:
  In1/1 -> Out1/1

== system VCU_CS75_12_30_test/长安CS75底盘程序，20ms一次/Input/DBC转化的messages（存底）/ReceiveMessages25/GW_3A2/SRS_RightRearBuckleSwitchSts_Sub ==
  In1 : Inport
  Out1 : Outport
  wires:
  In1/1 -> Out1/1

== system VCU_CS75_12_30_test/长安CS75底盘程序，20ms一次/Input/DBC转化的messages（存底）/ReceiveMessages25/GW_3A2/TCU_FailureLamp_Sub ==
  In1 : Inport
  Out1 : Outport
  wires:
  In1/1 -> Out1/1

== system VCU_CS75_12_30_test/长安CS75底盘程序，20ms一次/Input/DBC转化的messages（存底）/ReceiveMessages25/GW_3A2/TCU_GearForDisplay_Sub ==
  In1 : Inport
  Out1 : Outport
  wires:
  In1/1 -> Out1/1

== system VCU_CS75_12_30_test/长安CS75底盘程序，20ms一次/Input/DBC转化的messages（存底）/ReceiveMessages25/GW_3A2/TCU_GearIndication_Sub ==
  In1 : Inport
  Out1 : Outport
  wires:
  In1/1 -> Out1/1

== system VCU_CS75_12_30_test/长安CS75底盘程序，20ms一次/Input/DBC转化的messages（存底）/ReceiveMessages25/GW_3A2/TCU_PWRLamp_Sub ==
  In1 : Inport
  Out1 : Outport
  wires:
  In1/1 -> Out1/1

== system VCU_CS75_12_30_test/长安CS75底盘程序，20ms一次/Input/DBC转化的messages（存底）/ReceiveMessages25/GW_3A2/TCU_ReqTranTempWarning_Sub ==
  In1 : Inport
  Out1 : Outport
  wires:
  In1/1 -> Out1/1

== system VCU_CS75_12_30_test/长安CS75底盘程序，20ms一次/Input/DBC转化的messages（存底）/ReceiveMessages25/GW_3A2/TCU_WNTLamp_Sub ==
  In1 : Inport
  Out1 : Outport
  wires:
  In1/1 -> Out1/1

== system VCU_CS75_12_30_test/长安CS75底盘程序，20ms一次/Input/DBC转化的messages（存底）/ReceiveMessages26/GW_567/HU_Byroad_Sub ==
  In1 : Inport
  Out1 : Outport
  wires:
  In1/1 -> Out1/1

== system VCU_CS75_12_30_test/长安CS75底盘程序，20ms一次/Input/DBC转化的messages（存底）/ReceiveMessages26/GW_567/HU_EnterTunnelInfo_Sub ==
  In1 : Inport
  Out1 : Outport
  wires:
  In1/1 -> Out1/1

== system VCU_CS75_12_30_test/长安CS75底盘程序，20ms一次/Input/DBC转化的messages（存底）/ReceiveMessages26/GW_567/HU_NavGuiganceStatus_Sub ==
  In1 : Inport
  Out1 : Outport
  wires:
  In1/1 -> Out1/1

== system VCU_CS75_12_30_test/长安CS75底盘程序，20ms一次/Input/DBC转化的messages（存底）/ReceiveMessages26/GW_567/HU_TunnelDistance_Sub ==
  In1 : Inport
  Out1 : Outport
  wires:
  In1/1 -> Out1/1

== system VCU_CS75_12_30_test/长安CS75底盘程序，20ms一次/Input/DBC转化的messages（存底）/ReceiveMessages26/GW_567/HU_TunnelLength_Sub ==
  In1 : Inport
  Out1 : Outport
  wires:
  In1/1 -> Out1/1

== system VCU_CS75_12_30_test/长安CS75底盘程序，20ms一次/Input/DBC转化的messages（存底）/ReceiveMessages27/HU_GPS_500/GPSCurrentLocationValid_Sub ==
  In1 : Inport
  Out1 : Outport
  wires:
  In1/1 -> Out1/1

== system VCU_CS75_12_30_test/长安CS75底盘程序，20ms一次/Input/DBC转化的messages（存底）/ReceiveMessages28/LAS_36E/LAS_CheckSum_id36E_Sub ==
  In1 : Inport
  Out1 : Outport
  wires:
  In1/1 -> Out1/1

== system VCU_CS75_12_30_test/长安CS75底盘程序，20ms一次/Input/DBC转化的messages（存底）/ReceiveMessages28/LAS_36E/LAS_LaneEquationC1_Sub ==
  In1 : Inport
  Out1 : Outport
  wires:
  In1/1 -> Out1/1

== system VCU_CS75_12_30_test/长安CS75底盘程序，20ms一次/Input/DBC转化的messages（存底）/ReceiveMessages28/LAS_36E/LAS_LaneEquationC3_Sub ==
  In1 : Inport
  Out1 : Outport
  wires:
  In1/1 -> Out1/1

== system VCU_CS75_12_30_test/长安CS75底盘程序，20ms一次/Input/DBC转化的messages（存底）/ReceiveMessages28/LAS_36E/LAS_LaneEquationStatus_Sub ==
  In1 : Inport
  Out1 : Outport
  wires:
  In1/1 -> Out1/1

== system VCU_CS75_12_30_test/长安CS75底盘程序，20ms一次/Input/DBC转化的messages（存底）/ReceiveMessages28/LAS_36E/LAS_RoadCurvatureFar_Sub ==
  In1 : Inport
  Out1 : Outport
  wires:
  In1/1 -> Out1/1

== system VCU_CS75_12_30_test/长安CS75底盘程序，20ms一次/Input/DBC转化的messages（存底）/ReceiveMessages28/LAS_36E/LAS_RoadCurvatureNear_Sub ==
  In1 : Inport
  Out1 : Outport
  wires:
  In1/1 -> Out1/1

== system VCU_CS75_12_30_test/长安CS75底盘程序，20ms一次/Input/DBC转化的messages（存底）/ReceiveMessages28/LAS_36E/LAS_RollingCounter_id36E_Sub ==
  In1 : Inport
  Out1 : Outport
  wires:
  In1/1 -> Out1/1

== system VCU_CS75_12_30_test/长安CS75底盘程序，20ms一次/Input/DBC转化的messages（存底）/ReceiveMessages3/EMS_276/EMS_RealAccPedal_Sub ==
  In1 : Inport
  Out1 : Outport
  wires:
  In1/1 -> Out1/1

== system VCU_CS75_12_30_test/长安CS75底盘程序，20ms一次/Input/DBC转化的messages（存底）/ReceiveMessages4/EPB_256/EPB_Checksum_Sub ==
  In1 : Inport
  Out1 : Outport
  wires:
  In1/1 -> Out1/1

== system VCU_CS75_12_30_test/长安CS75底盘程序，20ms一次/Input/DBC转化的messages（存底）/ReceiveMessages4/EPB_256/EPB_FailStatus_Sub ==
  In1 : Inport
  Out1 : Outport
  wires:
  In1/1 -> Out1/1

== system VCU_CS75_12_30_test/长安CS75底盘程序，20ms一次/Input/DBC转化的messages（存底）/ReceiveMessages4/EPB_256/EPB_FailureLamp_Sub ==
  In1 : Inport
  Out1 : Outport
  wires:
  In1/1 -> Out1/1

== system VCU_CS75_12_30_test/长安CS75底盘程序，20ms一次/Input/DBC转化的messages（存底）/ReceiveMessages4/EPB_256/EPB_FunctionLamp_Sub ==
  In1 : Inport
  Out1 : Outport
  wires:
  In1/1 -> Out1/1

== system VCU_CS75_12_30_test/长安CS75底盘程序，20ms一次/Input/DBC转化的messages（存底）/ReceiveMessages4/EPB_256/EPB_RollingCounter_id256_Sub ==
  In1 : Inport
  Out1 : Outport
  wires:
  In1/1 -> Out1/1

== system VCU_CS75_12_30_test/长安CS75底盘程序，20ms一次/Input/DBC转化的messages（存底）/ReceiveMessages4/EPB_256/EPB_Status_Sub ==
  In1 : Inport
  Out1 : Outport
  wires:
  In1/1 -> Out1/1

== system VCU_CS75_12_30_test/长安CS75底盘程序，20ms一次/Input/DBC转化的messages（存底）/ReceiveMessages5/EPS_20A/EPS_APA_AbortFeedback_Sub ==
  In1 : Inport
  Out1 : Outport
  wires:
  In1/1 -> Out1/1

== system VCU_CS75_12_30_test/长安CS75底盘程序，20ms一次/Input/DBC转化的messages（存底）/ReceiveMessages5/EPS_20A/EPS_APA_ControlFeedback_Sub ==
  In1 : Inport
  Out1 : Outport
  wires:
  In1/1 -> Out1/1

== system VCU_CS75_12_30_test/长安CS75底盘程序，20ms一次/Input/DBC转化的messages（存底）/ReceiveMessages5/EPS_20A/EPS_APA_EpasFailed_Sub ==
  In1 : Inport
  Out1 : Outport
  wires:
  In1/1 -> Out1/1

== system VCU_CS75_12_30_test/长安CS75底盘程序，20ms一次/Input/DBC转化的messages（存底）/ReceiveMessages5/EPS_20A/EPS_Checksum_Sub ==
  In1 : Inport
  Out1 : Outport
  wires:
  In1/1 -> Out1/1

== system VCU_CS75_12_30_test/长安CS75底盘程序，20ms一次/Input/DBC转化的messages（存底）/ReceiveMessages5/EPS_20A/EPS_ConcussAvailabilityStatus_Sub ==
  In1 : Inport
  Out1 : Outport
  wires:
  In1/1 -> Out1/1

== system VCU_CS75_12_30_test/长安CS75底盘程序，20ms一次/Input/DBC转化的messages（存底）/ReceiveMessages5/EPS_20A/EPS_EPSFailed_Sub ==
  In1 : Inport
  Out1 : Outport
  wires:
  In1/1 -> Out1/1

== system VCU_CS75_12_30_test/长安CS75底盘程序，20ms一次/Input/DBC转化的messages（存底）/ReceiveMessages5/EPS_20A/EPS_RollingCounter_Sub ==
  In1 : Inport
  Out1 : Outport
  wires:
  In1/1 -> Out1/1

== system VCU_CS75_12_30_test/长安CS75底盘程序，20ms一次/Input/DBC转化的messages（存底）/ReceiveMessages5/EPS_20A/EPS_SteeringTorque_Sub ==
  In1 : Inport
  Out1 : Outport
  wires:
  In1/1 -> Out1/1

== system VCU_CS75_12_30_test/长安CS75底盘程序，20ms一次/Input/DBC转化的messages（存底）/ReceiveMessages5/EPS_20A/EPS_TorqueSensorStatus_Sub ==
  In1 : Inport
  Out1 : Outport
  wires:
  In1/1 -> Out1/1

== system VCU_CS75_12_30_test/长安CS75底盘程序，20ms一次/Input/DBC转化的messages（存底）/ReceiveMessages6/EPS_21A/CRC_Sub ==
  In1 : Inport
  Out1 : Outport
  wires:
  In1/1 -> Out1/1

== system VCU_CS75_12_30_test/长安CS75底盘程序，20ms一次/Input/DBC转化的messages（存底）/ReceiveMessages6/EPS_21A/EPS_AvailabilityStatus_Sub ==
  In1 : Inport
  Out1 : Outport
  wires:
  In1/1 -> Out1/1

== system VCU_CS75_12_30_test/长安CS75底盘程序，20ms一次/Input/DBC转化的messages（存底）/ReceiveMessages6/EPS_21A/EPS_IACC_abortReson_Sub ==
  In1 : Inport
  Out1 : Outport
  wires:
  In1/1 -> Out1/1

== system VCU_CS75_12_30_test/长安CS75底盘程序，20ms一次/Input/DBC转化的messages（存底）/ReceiveMessages6/EPS_21A/EPS_MeasTsionBatTorquevalid_Sub ==
  In1 : Inport
  Out1 : Outport
  wires:
  In1/1 -> Out1/1

== system VCU_CS75_12_30_test/长安CS75底盘程序，20ms一次/Input/DBC转化的messages（存底）/ReceiveMessages6/EPS_21A/EPS_MeasuredTosionBatTorque_Sub ==
  In1 : Inport
  Out1 : Outport
  wires:
  In1/1 -> Out1/1

== system VCU_CS75_12_30_test/长安CS75底盘程序，20ms一次/Input/DBC转化的messages（存底）/ReceiveMessages6/EPS_21A/Rollingcounter_Sub ==
  In1 : Inport
  Out1 : Outport
  wires:
  In1/1 -> Out1/1

== system VCU_CS75_12_30_test/长安CS75底盘程序，20ms一次/Input/DBC转化的messages（存底）/ReceiveMessages7/ESP_277/ESP_ABAactive_Sub ==
  In1 : Inport
  Out1 : Outport
  wires:
  In1/1 -> Out1/1

== system VCU_CS75_12_30_test/长安CS75底盘程序，20ms一次/Input/DBC转化的messages（存底）/ReceiveMessages7/ESP_277/ESP_ABAavailable_Sub ==
  In1 : Inport
  Out1 : Outport
  wires:
  In1/1 -> Out1/1

== system VCU_CS75_12_30_test/长安CS75底盘程序，20ms一次/Input/DBC转化的messages（存底）/ReceiveMessages7/ESP_277/ESP_AEBAvailable_Sub ==
  In1 : Inport
  Out1 : Outport
  wires:
  In1/1 -> Out1/1

== system VCU_CS75_12_30_test/长安CS75底盘程序，20ms一次/Input/DBC转化的messages（存底）/ReceiveMessages7/ESP_277/ESP_AEBdecActive_Sub ==
  In1 : Inport
  Out1 : Outport
  wires:
  In1/1 -> Out1/1

== system VCU_CS75_12_30_test/长安CS75底盘程序，20ms一次/Input/DBC转化的messages（存底）/ReceiveMessages7/ESP_277/ESP_AWBactive_Sub ==
  In1 : Inport
  Out1 : Outport
  wires:
  In1/1 -> Out1/1

== system VCU_CS75_12_30_test/长安CS75底盘程序，20ms一次/Input/DBC转化的messages（存底）/ReceiveMessages7/ESP_277/ESP_AWBavailable_Sub ==
  In1 : Inport
  Out1 : Outport
  wires:
  In1/1 -> Out1/1

== system VCU_CS75_12_30_test/长安CS75底盘程序，20ms一次/Input/DBC转化的messages（存底）/ReceiveMessages7/ESP_277/ESP_BrakeForce_Sub ==
  In1 : Inport
  Out1 : Outport
  wires:
  In1/1 -> Out1/1

== system VCU_CS75_12_30_test/长安CS75底盘程序，20ms一次/Input/DBC转化的messages（存底）/ReceiveMessages7/ESP_277/ESP_BrakeOverHeat_Sub ==
  In1 : Inport
  Out1 : Outport
  wires:
  In1/1 -> Out1/1

== system VCU_CS75_12_30_test/长安CS75底盘程序，20ms一次/Input/DBC转化的messages（存底）/ReceiveMessages7/ESP_277/ESP_CDD_Active_APA_Sub ==
  In1 : Inport
  Out1 : Outport
  wires:
  In1/1 -> Out1/1

== system VCU_CS75_12_30_test/长安CS75底盘程序，20ms一次/Input/DBC转化的messages（存底）/ReceiveMessages7/ESP_277/ESP_CDD_Active_Sub ==
  In1 : Inport
  Out1 : Outport
  wires:
  In1/1 -> Out1/1

== system VCU_CS75_12_30_test/长安CS75底盘程序，20ms一次/Input/DBC转化的messages（存底）/ReceiveMessages7/ESP_277/ESP_CDD_Available_APA_Sub ==
  In1 : Inport
  Out1 : Outport
  wires:
  In1/1 -> Out1/1

== system VCU_CS75_12_30_test/长安CS75底盘程序，20ms一次/Input/DBC转化的messages（存底）/ReceiveMessages7/ESP_277/ESP_CDD_Available_Sub ==
  In1 : Inport
  Out1 : Outport
  wires:
  In1/1 -> Out1/1

== system VCU_CS75_12_30_test/长安CS75底盘程序，20ms一次/Input/DBC转化的messages（存底）/ReceiveMessages7/ESP_277/ESP_CheckSum_277_Sub ==
  In1 : Inport
  Out1 : Outport
  wires:
  In1/1 -> Out1/1

== system VCU_CS75_12_30_test/长安CS75底盘程序，20ms一次/Input/DBC转化的messages（存底）/ReceiveMessages7/ESP_277/ESP_PrefillActive_Sub ==
  In1 : Inport
  Out1 : Outport
  wires:
  In1/1 -> Out1/1

== system VCU_CS75_12_30_test/长安CS75底盘程序，20ms一次/Input/DBC转化的messages（存底）/ReceiveMessages7/ESP_277/ESP_PrefillAvailable_Sub ==
  In1 : Inport
  Out1 : Outport
  wires:
  In1/1 -> Out1/1

== system VCU_CS75_12_30_test/长安CS75底盘程序，20ms一次/Input/DBC转化的messages（存底）/ReceiveMessages7/ESP_277/ESP_RollingCounter_277_Sub ==
  In1 : Inport
  Out1 : Outport
  wires:
  In1/1 -> Out1/1

== system VCU_CS75_12_30_test/长安CS75底盘程序，20ms一次/Input/DBC转化的messages（存底）/ReceiveMessages7/ESP_277/ESP_TCSActive_Sub ==
  In1 : Inport
  Out1 : Outport
  wires:
  In1/1 -> Out1/1

== system VCU_CS75_12_30_test/长安CS75底盘程序，20ms一次/Input/DBC转化的messages（存底）/ReceiveMessages7/ESP_277/ESP_VDCActive_Sub ==
  In1 : Inport
  Out1 : Outport
  wires:
  In1/1 -> Out1/1

== system VCU_CS75_12_30_test/长安CS75底盘程序，20ms一次/Input/DBC转化的messages（存底）/ReceiveMessages7/ESP_277/ESP_VehicleStandstill_Sub ==
  In1 : Inport
  Out1 : Outport
  wires:
  In1/1 -> Out1/1

== system VCU_CS75_12_30_test/长安CS75底盘程序，20ms一次/Input/DBC转化的messages（存底）/ReceiveMessages8/ESP_280/Wheel_Speed_FL_Data_Sub ==
  In1 : Inport
  Out1 : Outport
  wires:
  In1/1 -> Out1/1

== system VCU_CS75_12_30_test/长安CS75底盘程序，20ms一次/Input/DBC转化的messages（存底）/ReceiveMessages8/ESP_280/Wheel_Speed_FL_Direction_Sub ==
  In1 : Inport
  Out1 : Outport
  wires:
  In1/1 -> Out1/1

== system VCU_CS75_12_30_test/长安CS75底盘程序，20ms一次/Input/DBC转化的messages（存底）/ReceiveMessages8/ESP_280/Wheel_Speed_FL_Valid_Data_Sub ==
  In1 : Inport
  Out1 : Outport
  wires:
  In1/1 -> Out1/1

== system VCU_CS75_12_30_test/长安CS75底盘程序，20ms一次/Input/DBC转化的messages（存底）/ReceiveMessages8/ESP_280/Wheel_Speed_FR_Data_Sub ==
  In1 : Inport
  Out1 : Outport
  wires:
  In1/1 -> Out1/1

== system VCU_CS75_12_30_test/长安CS75底盘程序，20ms一次/Input/DBC转化的messages（存底）/ReceiveMessages8/ESP_280/Wheel_Speed_FR_Direction_Sub ==
  In1 : Inport
  Out1 : Outport
  wires:
  In1/1 -> Out1/1

== system VCU_CS75_12_30_test/长安CS75底盘程序，20ms一次/Input/DBC转化的messages（存底）/ReceiveMessages8/ESP_280/Wheel_Speed_FR_Valid_Data_Sub ==
  In1 : Inport
  Out1 : Outport
  wires:
  In1/1 -> Out1/1

== system VCU_CS75_12_30_test/长安CS75底盘程序，20ms一次/Input/DBC转化的messages（存底）/ReceiveMessages8/ESP_280/Wheel_Speed_RL_Data_Sub ==
  In1 : Inport
  Out1 : Outport
  wires:
  In1/1 -> Out1/1
